simulink model "Coefficients"  (R2024b)
settings: Solver=VariableStepAuto  StartTime=0.0  StopTime=10.0  RelTol=1e-3
values from neighbouring files (symbols this model uses):
  b = params.b    [Aerodynamics_Coefficient.m]    (also in AeroforcesandMoments.m; initACFT_high.m = 21; initACFT_low.m = 21; init_Cessna.m = 10.9728)
  c = params.c    [Aerodynamics_Coefficient.m]    (also in AeroforcesandMoments.m; initACFT_high.m = 2.5; initACFT_low.m = 2.5; init_Cessna.m = 1.49352)
  CD0 = params.CD0    [Aerodynamics_Coefficient.m]    (also in initACFT_high.m = 0.0281; initACFT_low.m = 0.023; init_Cessna.m = 0.027)
  CD_alpha = params.CD_alpha    [Aerodynamics_Coefficient.m]    (also in initACFT_high.m = 0.5157; initACFT_low.m = 0.1318; init_Cessna.m = 0.26)
  CD_elev = params.CD_elev    [Aerodynamics_Coefficient.m]    (also in initACFT_high.m = 0.0178; initACFT_low.m = 0.0178; init_Cessna.m = 0)
  CI_beta = params.CI_beta    [Aerodynamics_Coefficient.m]
  CI_p = params.CI_p    [Aerodynamics_Coefficient.m]
  CI_r = params.CI_r    [Aerodynamics_Coefficient.m]
  CI_rud = params.CI_rud    [Aerodynamics_Coefficient.m]
  CL0 = params.CL0    [Aerodynamics_Coefficient.m]    (also in initACFT_high.m = 0.209; initACFT_low.m = 0.19; init_Cessna.m = 0.307)
  CL_alpha = params.CL_alpha    [Aerodynamics_Coefficient.m]    (also in initACFT_high.m = 8.7491; initACFT_low.m = 6.1879; init_Cessna.m = 4.41)
  CL_elev = params.CL_elev    [Aerodynamics_Coefficient.m]    (also in initACFT_high.m = 0.538; initACFT_low.m = 0.4727; init_Cessna.m = 0.43)
  CL_q = params.CL_q    [Aerodynamics_Coefficient.m]    (also in initACFT_high.m = 4.14; initACFT_low.m = 4.66; init_Cessna.m = 3.9)
  Cm0 = params.Cm0    [Aerodynamics_Coefficient.m]    (also in initACFT_high.m = 0; initACFT_low.m = 0.0133; init_Cessna.m = 0.04)
  Cm_alpha = params.Cm_alpha    [Aerodynamics_Coefficient.m]    (also in initACFT_high.m = -2.4351; initACFT_low.m = -2.0168; init_Cessna.m = -0.613)
  Cm_AlphaDot = params.Cm_AlphaDot    [Aerodynamics_Coefficient.m]    (also in initACFT_high.m = -4.53; initACFT_low.m = -6.76; init_Cessna.m = -7.27)
  Cm_elev = params.Cm_elev    [Aerodynamics_Coefficient.m]    (also in initACFT_high.m = -1.9079; initACFT_low.m = -1.6788; init_Cessna.m = -1.122)
  Cm_q = params.Cm_q    [Aerodynamics_Coefficient.m]    (also in initACFT_high.m = -37.6; initACFT_low.m = -36.3; init_Cessna.m = -12.4)
  Cn_ail = -8.5944e-04    (= -0.00085944)    [initACFT_high.m]    (also in initACFT_low.m = -0.00063025; init_Cessna.m = -0.0216)
  Cn_beta = 0.1478    [initACFT_high.m]    (also in initACFT_low.m = 0.1209; init_Cessna.m = 0.0587)
  Cn_p = -0.114    [initACFT_high.m]    (also in initACFT_low.m; init_Cessna.m = -0.0278)
  Cn_r = -0.15    [initACFT_high.m]    (also in initACFT_low.m = -0.3; init_Cessna.m = -0.0937)
  Cn_rud = -0.1100    (= -0.11)    [initACFT_high.m]    (also in initACFT_low.m = -0.102; init_Cessna.m = -0.0645)
  CY_ail = 0    [initACFT_high.m]    (also in initACFT_low.m; init_Cessna.m)
  CY_beta = params.CY_beta    [Aerodynamics_Coefficient.m]    (also in initACFT_high.m = -1.2777; initACFT_low.m = -1.1803; init_Cessna.m = -0.404)
  CY_p = params.CY_p    [Aerodynamics_Coefficient.m]    (also in initACFT_high.m = 0.3; initACFT_low.m = 0.3; init_Cessna.m = -0.075)
  CY_r = params.CY_r    [Aerodynamics_Coefficient.m]    (also in initACFT_high.m = 0.91; initACFT_low.m = 0.91; init_Cessna.m = 0.214)
  CY_rud = params.CY_rud    [Aerodynamics_Coefficient.m]    (also in initACFT_high.m = 0.4343; initACFT_low.m = 0.4016; init_Cessna.m = 0.187)
  S = 45    [initACFT_high.m]    (also in initACFT_low.m; init_Cessna.m = 16.2)
undefined symbols (not defined in the file or in its folder): CI_ail, CL_AlphaDot_, Y_cg, Z_cg

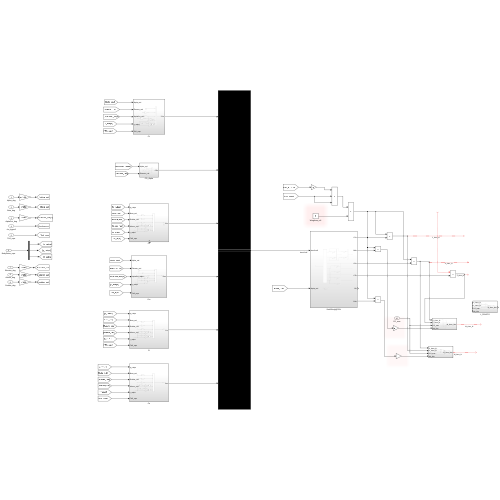
[thumbnail: Simulink's stored preview of the top-level diagram]
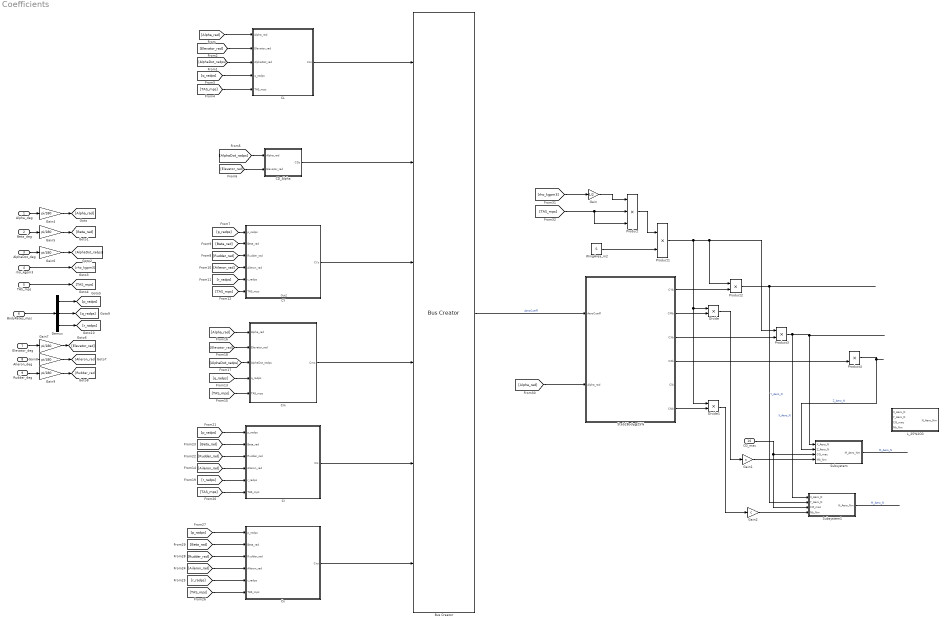
== system Coefficients ==
  Alpha_deg : Inport
  Beta_deg : Inport  Port=2
  AlphaDot_deg : Inport  Port=3
  rho_kgpm3 : Inport  Port=4
  TAS_mps : Inport  Port=5
  BodyRates_mps : Inport  Port=6
  Elevator_deg : Inport  Port=7
  Aileron_deg : Inport  Port=8
  Rudder_deg : Inport  Port=9
  CG_mac : Inport  Port=10
  Bus Creator : BusCreator  Inputs=6
  CD_Alpha : Subsystem
  CI : Subsystem
  CL : Subsystem
  CY : Subsystem
      settings: PortSchema="{\"entries\":[{\"content\":{\"sides\":[{\"content\":{\"connectorIds\":[\"In1\",\"In2\",\"In3\",\"In4\",\"In5\",\"In6\"]},\"type\":\"ConnectorPlacement.EquallySpacedRectSide\",\"uuid\":\"cf27de7d-07f8-4cbf-b6d7-bb20821c77c6\"},{\"content\":{\"connectorIds\":[\"Out1\"],\"side\":\"RIGHT\"},\"type\":\"ConnectorPlacement.EquallySpacedRectSide\",\"uuid\":\"f24d40b1-0b9f-4cab-b37e-a7503e974de5\"},{\"content\":{\"side\":\"TOP\"},\"type\":\"ConnectorPlacement.EquallySpacedRectSide\",\"uuid\":\"b0626d26-2b97-4927-834a-53d4ff987b45\"},{\"content\":{\"connectorIds\":[\"Out2\"],\"side\":\"BOTTOM\"},\"type\":\"ConnectorPlacement.EquallySpacedRectSide\",\"uuid\":\"9cececd4-1f67-47fb-9396-7a7e586ce31d\"}]},\"type\":\"ConnectorPlacement.EquallySpacedConnector\",\"uuid\":\"f6062f6f-5301-4f2b-96bc-d3beb1582379\"}],\"packageUris\":[\"http://schema.mathworks.com/mf0/Connector/R2020b\"],\"version\":\"1.0\"}"
  Cm : Subsystem
  Cn : Subsystem
  Demux : Demux  Outputs=3
  Divide : Product
  Divide1 : Product
  Gain : Gain  Gain=1/2
  Gain1 : Gain  Gain=c
  Gain2 : Gain  Gain=c
  Gain{4..9} (6 alike) : Gain  Gain=pi/180
  L_25%2CG : Subsystem
  Product : Product  Inputs=3
  Product{1..4} (4 alike) : Product
  Stab2Body@25% : Subsystem
  Subsystem : Subsystem
  Subsystem1 : Subsystem
  WingArea_m2 : Constant  Value=S
  wires:
  AlphaDot_deg/1 -> Gain6/1
  rho_kgpm3/1 -> [rho_kgpm3]
  TAS_mps/1 -> [TAS_mps]
  Elevator_deg/1 -> Gain7/1
  Aileron_deg/1 -> Gain8/1
  Rudder_deg/1 -> Gain9/1
  Alpha_deg/1 -> Gain4/1
  Gain4/1 -> [Alpha_rad]
  Beta_deg/1 -> Gain5/1
  Gain5/1 -> [Beta_rad]
  Gain6/1 -> [AlphaDot_radps]
  Gain7/1 -> [Elevator_rad]
  Gain8/1 -> [Aileron_rad]
  Gain9/1 -> [Rudder_rad]
  [Elevator_rad] -> CL/2(Elevator_rad)
  [Alpha_rad] -> CL/1(Alpha_rad)
  [AlphaDot_radps] -> CL/3(AlphaDot_rad)
  [q_radps] -> CL/4(q_radps)
  BodyRates_mps/1 -> Demux/1
  Demux/2 -> [q_radps]
  Demux/1 -> [p_radps]
  Demux/3 -> [r_radps]
  [TAS_mps] -> CL/5(TAS_mps)
  [Elevator_rad] -> CD_Alpha/2(Elevator_rad)
  [AlphaDot_radps] -> CD_Alpha/1(Alpha_rad)
  [p_radps] -> CY/1(p_radps)
  [Rudder_rad] -> CY/3(Rudder_rad)
  [Beta_rad] -> CY/2(Beta_rad)
  [Aileron_rad] -> CY/4(Aileron_rad)
  [r_radps] -> CY/5(r_radps)
  [TAS_mps] -> CY/6(TAS_mps)
  [TAS_mps] -> Cm/5(TAS_mps)
  [Alpha_rad] -> Cm/1(Alpha_rad)
  [Elevator_rad] -> Cm/2(Elevator_rad)
  [AlphaDot_radps] -> Cm/3(AlphaDot_radps)
  [q_radps] -> Cm/4(q_radps)
  [p_radps] -> CI/1(p_radps)
  [Beta_rad] -> CI/2(Beta_rad)
  [Rudder_rad] -> CI/3(Rudder_rad)
  [Aileron_rad] -> CI/4(Aileron_rad)
  [r_radps] -> CI/5(r_radps)
  [TAS_mps] -> CI/6(TAS_mps)
  [TAS_mps] -> Cn/6(TAS_mps)
  [r_radps] -> Cn/5(r_radps)
  [Aileron_rad] -> Cn/4(Aileron_rad)
  [Beta_rad] -> Cn/2(Beta_rad)
  [p_radps] -> Cn/1(p_radps)
  [Rudder_rad] -> Cn/3(Rudder_rad)
  CL/1(CLs) -> Bus Creator/1
  CD_Alpha/1(CDs) -> Bus Creator/2
  CY/1(CYs) -> Bus Creator/3
  Cm/1(Cms) -> Bus Creator/4
  CI/1(CIs) -> Bus Creator/5
  Cn/1(Cns) -> Bus Creator/6
  Bus Creator/1 -> Stab2Body@25%/1(AeroCoeff)  "AeroCoeff"
  [Alpha_rad] -> Stab2Body@25%/2(Alpha_rad)
  [rho_kgpm3] -> Gain/1
  Gain/1 -> Product/1
  [TAS_mps] -> Product/3, Product/2
  WingArea_m2/1 -> Product1/2
  Product/1 -> Product1/1
  Stab2Body@25%/1(CYb) -> Product2/2
  Stab2Body@25%/3(CXb) -> Product3/2
  Stab2Body@25%/4(CZb) -> Product4/2
  Product1/1 -> Divide1/1, Divide/1, Product2/1, Product3/1
  ? -> Product4/1
  Product2/1 -> Subsystem1/2(Y_Aero_N)  "Y_Aero_N"
  Product3/1 -> Subsystem1/1(X_Aero_N), Subsystem/1(X_Aero_N)  "X_Aero_N"
  Product4/1 -> Subsystem/2(Z_Aero_N)  "Z_Aero_N"
  CG_mac/1 -> Subsystem1/3(CG_mac), Subsystem/3(CG_mac)
  Stab2Body@25%/2(CMb) -> Divide/2
  Divide/1 -> Gain1/1
  Subsystem/1(M_Aero_Nm) -> ?  "M_Aero_N"
  Gain1/1 -> Subsystem/4(Mb_Nm)
  Subsystem1/1(N_Aero_Nm) -> ?  "M_Aero_N"
  Stab2Body@25%/6(CNb) -> Divide1/2
  Gain2/1 -> Subsystem1/4(Nb_Nm)
  Divide1/1 -> Gain2/1

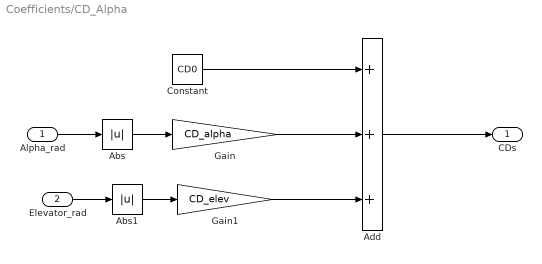
== system Coefficients/CD_Alpha ==
  Alpha_rad : Inport
  Elevator_rad : Inport  Port=2
  Abs : Abs  SaturateOnIntegerOverflow=off
  Abs1 : Abs  SaturateOnIntegerOverflow=off
  Add : Sum  Inputs=+++
  Constant : Constant  Value=CD0
  Gain : Gain  Gain=CD_alpha
  Gain1 : Gain  Gain=CD_elev
  CDs : Outport
  wires:
  Abs1/1 -> Gain1/1
  Alpha_rad/1 -> Abs/1
  Constant/1 -> Add/1
  Abs/1 -> Gain/1
  Add/1 -> CDs/1
  Elevator_rad/1 -> Abs1/1
  Gain1/1 -> Add/3
  Gain/1 -> Add/2

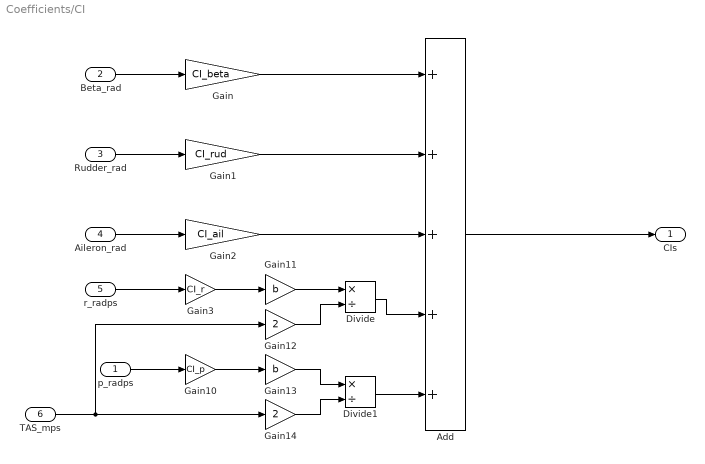
== system Coefficients/CI ==
  p_radps : Inport
  Beta_rad : Inport  Port=2
  Rudder_rad : Inport  Port=3
  Aileron_rad : Inport  Port=4
  r_radps : Inport  Port=5
  TAS_mps : Inport  Port=6
  Add : Sum  Inputs=+++++
  Divide : Product  Inputs=*/
  Divide1 : Product  Inputs=*/
  Gain : Gain  Gain=CI_beta
  Gain1 : Gain  Gain=CI_rud
  Gain10 : Gain  Gain=CI_p
  Gain11 : Gain  Gain=b
  Gain12 : Gain  Gain=2
  Gain13 : Gain  Gain=b
  Gain14 : Gain  Gain=2
  Gain2 : Gain  Gain=CI_ail
  Gain3 : Gain  Gain=CI_r
  CIs : Outport
  wires:
  Gain13/1 -> Divide1/1
  Gain/1 -> Add/1
  Gain3/1 -> Gain11/1
  Rudder_rad/1 -> Gain1/1
  Gain2/1 -> Add/3
  Add/1 -> CIs/1
  Gain12/1 -> Divide/2
  Gain11/1 -> Divide/1
  Gain14/1 -> Divide1/2
  TAS_mps/1 -> Gain12/1, Gain14/1
  Gain10/1 -> Gain13/1
  Divide/1 -> Add/4
  p_radps/1 -> Gain10/1
  Gain1/1 -> Add/2
  Aileron_rad/1 -> Gain2/1
  Beta_rad/1 -> Gain/1
  r_radps/1 -> Gain3/1
  Divide1/1 -> Add/5

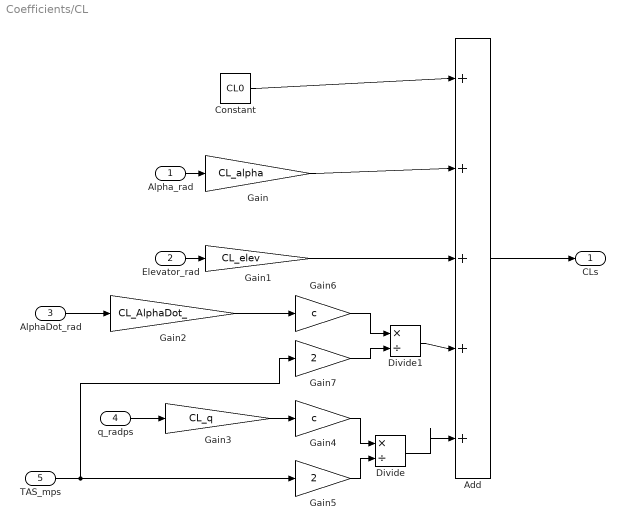
== system Coefficients/CL ==
  Alpha_rad : Inport
  Elevator_rad : Inport  Port=2
  AlphaDot_rad : Inport  Port=3
  q_radps : Inport  Port=4
  TAS_mps : Inport  Port=5
  Add : Sum  Inputs=+++++
  Constant : Constant  Value=CL0
  Divide : Product  Inputs=*/
  Divide1 : Product  Inputs=*/
  Gain : Gain  Gain=CL_alpha
  Gain1 : Gain  Gain=CL_elev
  Gain2 : Gain  Gain=CL_AlphaDot_
  Gain3 : Gain  Gain=CL_q
  Gain4 : Gain  Gain=c
  Gain5 : Gain  Gain=2
  Gain6 : Gain  Gain=c
  Gain7 : Gain  Gain=2
  CLs : Outport
  wires:
  Alpha_rad/1 -> Gain/1
  q_radps/1 -> Gain3/1
  AlphaDot_rad/1 -> Gain2/1
  Gain1/1 -> Add/3
  Elevator_rad/1 -> Gain1/1
  Gain/1 -> Add/2
  Constant/1 -> Add/1
  Gain2/1 -> Gain6/1
  Add/1 -> CLs/1
  Gain3/1 -> Gain4/1
  TAS_mps/1 -> Gain7/1, Gain5/1
  Gain5/1 -> Divide/2
  Divide/1 -> Add/5
  Gain4/1 -> Divide/1
  Gain6/1 -> Divide1/1
  Divide1/1 -> Add/4
  Gain7/1 -> Divide1/2

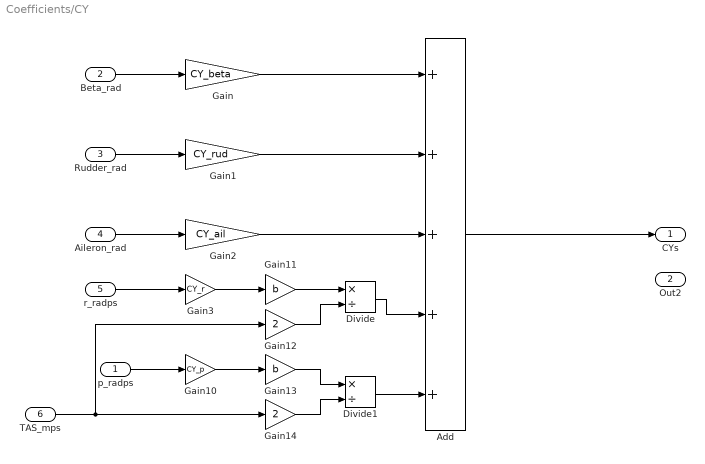
== system Coefficients/CY ==
  p_radps : Inport
  Beta_rad : Inport  Port=2
  Rudder_rad : Inport  Port=3
  Aileron_rad : Inport  Port=4
  r_radps : Inport  Port=5
  TAS_mps : Inport  Port=6
  Add : Sum  Inputs=+++++
  Divide : Product  Inputs=*/
  Divide1 : Product  Inputs=*/
  Gain : Gain  Gain=CY_beta
  Gain1 : Gain  Gain=CY_rud
  Gain10 : Gain  Gain=CY_p
  Gain11 : Gain  Gain=b
  Gain12 : Gain  Gain=2
  Gain13 : Gain  Gain=b
  Gain14 : Gain  Gain=2
  Gain2 : Gain  Gain=CY_ail
  Gain3 : Gain  Gain=CY_r
  CYs : Outport
  Out2 : Outport  Port=2
  wires:
  Gain13/1 -> Divide1/1
  Gain/1 -> Add/1
  Gain3/1 -> Gain11/1
  Rudder_rad/1 -> Gain1/1
  Gain2/1 -> Add/3
  Add/1 -> CYs/1
  Gain12/1 -> Divide/2
  Gain11/1 -> Divide/1
  Gain14/1 -> Divide1/2
  TAS_mps/1 -> Gain12/1, Gain14/1
  Gain10/1 -> Gain13/1
  Divide/1 -> Add/4
  p_radps/1 -> Gain10/1
  Gain1/1 -> Add/2
  Aileron_rad/1 -> Gain2/1
  Beta_rad/1 -> Gain/1
  r_radps/1 -> Gain3/1
  Divide1/1 -> Add/5

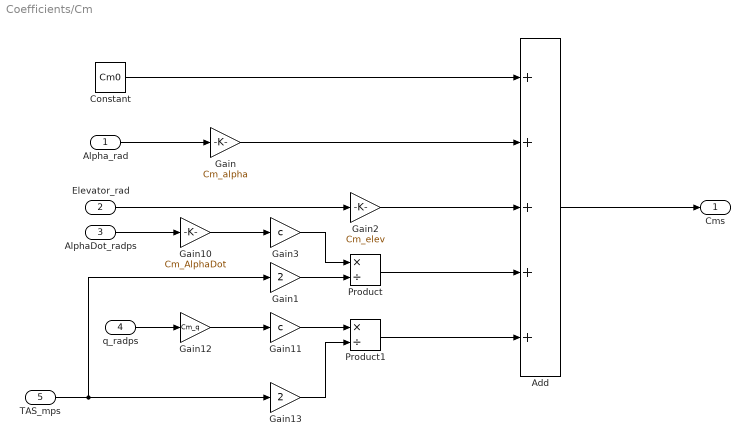
== system Coefficients/Cm ==
  Alpha_rad : Inport
  Elevator_rad : Inport  Port=2
  AlphaDot_radps : Inport  Port=3
  q_radps : Inport  Port=4
  TAS_mps : Inport  Port=5
  Add : Sum  Inputs=+++++
  Constant : Constant  Value=Cm0
  Gain : Gain  Gain=Cm_alpha
  Gain1 : Gain  Gain=2
  Gain10 : Gain  Gain=Cm_AlphaDot
  Gain11 : Gain  Gain=c
  Gain12 : Gain  Gain=Cm_q
  Gain13 : Gain  Gain=2
  Gain2 : Gain  Gain=Cm_elev
  Gain3 : Gain  Gain=c
  Product : Product  Inputs=*/
  Product1 : Product  Inputs=*/
  Cms : Outport
  wires:
  AlphaDot_radps/1 -> Gain10/1
  Elevator_rad/1 -> Gain2/1
  Constant/1 -> Add/1
  TAS_mps/1 -> Gain1/1, Gain13/1
  Gain1/1 -> Product/2
  Gain2/1 -> Add/3
  Alpha_rad/1 -> Gain/1
  Product1/1 -> Add/5
  Gain3/1 -> Product/1
  Gain13/1 -> Product1/2
  Gain12/1 -> Gain11/1
  q_radps/1 -> Gain12/1
  Gain10/1 -> Gain3/1
  Gain11/1 -> Product1/1
  Gain/1 -> Add/2
  Product/1 -> Add/4
  Add/1 -> Cms/1

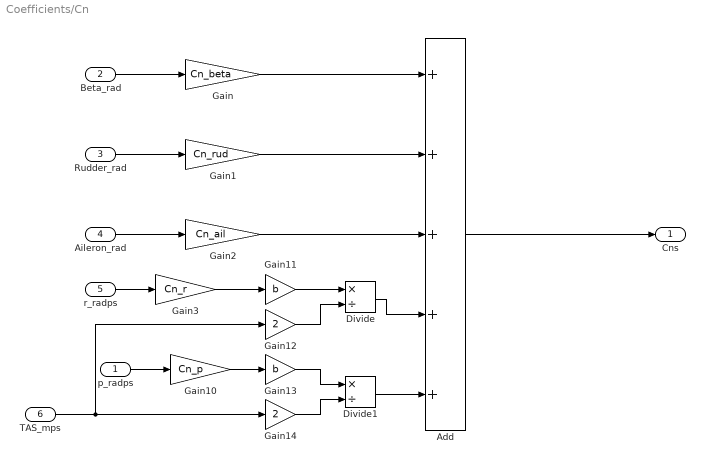
== system Coefficients/Cn ==
  p_radps : Inport
  Beta_rad : Inport  Port=2
  Rudder_rad : Inport  Port=3
  Aileron_rad : Inport  Port=4
  r_radps : Inport  Port=5
  TAS_mps : Inport  Port=6
  Add : Sum  Inputs=+++++
  Divide : Product  Inputs=*/
  Divide1 : Product  Inputs=*/
  Gain : Gain  Gain=Cn_beta
  Gain1 : Gain  Gain=Cn_rud
  Gain10 : Gain  Gain=Cn_p
  Gain11 : Gain  Gain=b
  Gain12 : Gain  Gain=2
  Gain13 : Gain  Gain=b
  Gain14 : Gain  Gain=2
  Gain2 : Gain  Gain=Cn_ail
  Gain3 : Gain  Gain=Cn_r
  Cns : Outport
  wires:
  Gain13/1 -> Divide1/1
  Gain/1 -> Add/1
  Gain3/1 -> Gain11/1
  Rudder_rad/1 -> Gain1/1
  Gain2/1 -> Add/3
  Add/1 -> Cns/1
  Gain12/1 -> Divide/2
  Gain11/1 -> Divide/1
  Gain14/1 -> Divide1/2
  TAS_mps/1 -> Gain12/1, Gain14/1
  Gain10/1 -> Gain13/1
  Divide/1 -> Add/4
  p_radps/1 -> Gain10/1
  Gain1/1 -> Add/2
  Aileron_rad/1 -> Gain2/1
  Beta_rad/1 -> Gain/1
  r_radps/1 -> Gain3/1
  Divide1/1 -> Add/5

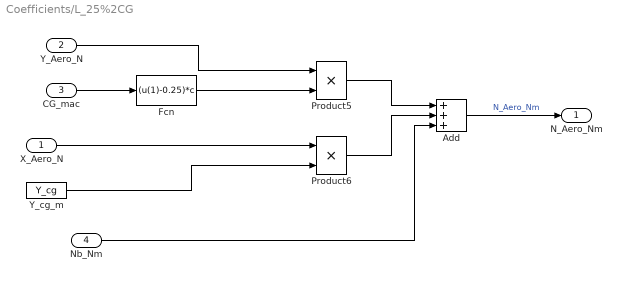
== system Coefficients/L_25%2CG ==
  X_Aero_N : Inport
  Y_Aero_N : Inport  Port=2
  CG_mac : Inport  Port=3
  Nb_Nm : Inport  Port=4
  Add : Sum  Inputs=+++
  Fcn : Fcn  Expr=(u(1)-0.25)*c
  Product5 : Product
  Product6 : Product
  Y_cg_m : Constant  Value=Y_cg
  N_Aero_Nm : Outport
  wires:
  Product6/1 -> Add/2
  CG_mac/1 -> Fcn/1
  Product5/1 -> Add/1
  Y_cg_m/1 -> Product6/2
  Y_Aero_N/1 -> Product5/1
  Fcn/1 -> Product5/2
  X_Aero_N/1 -> Product6/1
  Add/1 -> N_Aero_Nm/1  "N_Aero_Nm"
  Nb_Nm/1 -> Add/3

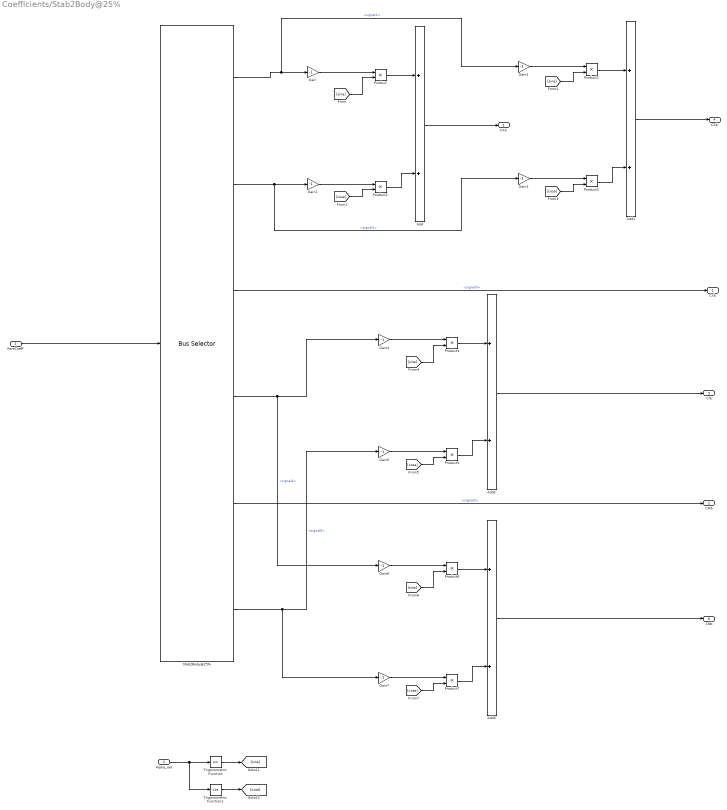
== system Coefficients/Stab2Body@25% ==
  AeroCoeff : Inport
  Alpha_rad : Inport  Port=2
  Add{,1..3} (4 alike) : Sum
  Gain{,1..7} (8 alike) : Gain  Gain=-1
  Product{,1..7} (8 alike) : Product
  Stab2Body@25% : BusSelector  OutputSignals=signal1,signal2,signal3,signal4,signal5,signal6
  Trigonometric Function : Trigonometry
  Trigonometric Function1 : Trigonometry  Operator=cos
  CYb : Outport
  CMb : Outport  Port=2
  CXb : Outport  Port=3
  CZb : Outport  Port=4
  Clb : Outport  Port=5
  CNb : Outport  Port=6
  wires:
  AeroCoeff/1 -> Stab2Body@25%/1
  Stab2Body@25%/5 -> CMb/1  "<signal5>"
  Stab2Body@25%/3 -> CYb/1  "<signal3>"
  Stab2Body@25%/1 -> Gain2/1, Gain/1  "<signal1>"
  Trigonometric Function/1 -> [sina]
  Trigonometric Function1/1 -> [cosa]
  Alpha_rad/1 -> Trigonometric Function1/1, Trigonometric Function/1
  Product/1 -> Add/1
  Product1/1 -> Add/2
  Gain/1 -> Product/1
  Gain1/1 -> Product1/1
  [sina] -> Product/2
  [cosa] -> Product1/2
  Add/1 -> CXb/1
  Product2/1 -> Add1/1
  Gain3/1 -> Product3/1
  [sina] -> Product2/2
  Add1/1 -> CZb/1
  Product3/1 -> Add1/2
  Gain2/1 -> Product2/1
  Stab2Body@25%/2 -> Gain3/1, Gain1/1  "<signal2>"
  [cosa] -> Product3/2
  Product4/1 -> Add2/1
  Gain5/1 -> Product5/1
  [sina] -> Product4/2
  Add2/1 -> Clb/1
  Stab2Body@25%/6 -> Gain7/1, Gain5/1  "<signal6>"
  Product5/1 -> Add2/2
  Stab2Body@25%/4 -> Gain6/1, Gain4/1  "<signal4>"
  Gain4/1 -> Product4/1
  [cosa] -> Product5/2
  [sina] -> Product6/2
  Gain6/1 -> Product6/1
  [cosa] -> Product7/2
  Gain7/1 -> Product7/1
  Add3/1 -> CNb/1
  Product6/1 -> Add3/1
  Product7/1 -> Add3/2

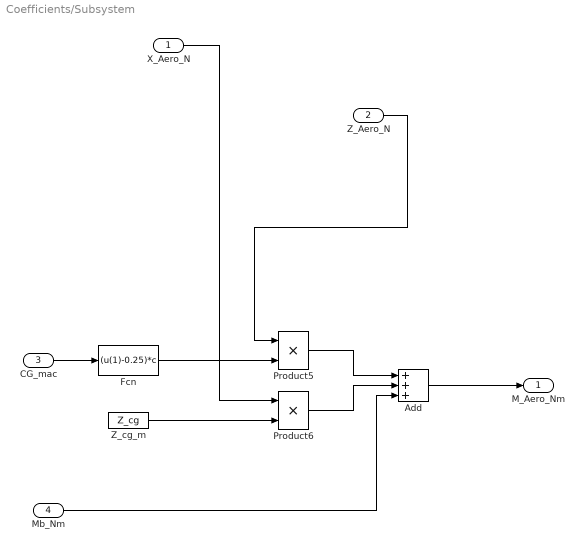
== system Coefficients/Subsystem ==
  X_Aero_N : Inport
  Z_Aero_N : Inport  Port=2
  CG_mac : Inport  Port=3
  Mb_Nm : Inport  Port=4
  Add : Sum  Inputs=+++
  Fcn : Fcn  Expr=(u(1)-0.25)*c
  Product5 : Product
  Product6 : Product
  Z_cg_m : Constant  Value=Z_cg
  M_Aero_Nm : Outport
  wires:
  Product6/1 -> Add/2
  CG_mac/1 -> Fcn/1
  Product5/1 -> Add/1
  Z_cg_m/1 -> Product6/2
  Z_Aero_N/1 -> Product5/1
  Fcn/1 -> Product5/2
  X_Aero_N/1 -> Product6/1
  Add/1 -> M_Aero_Nm/1
  Mb_Nm/1 -> Add/3

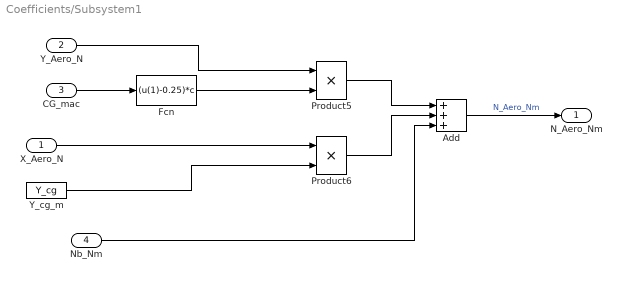
== system Coefficients/Subsystem1 ==
  X_Aero_N : Inport
  Y_Aero_N : Inport  Port=2
  CG_mac : Inport  Port=3
  Nb_Nm : Inport  Port=4
  Add : Sum  Inputs=+++
  Fcn : Fcn  Expr=(u(1)-0.25)*c
  Product5 : Product
  Product6 : Product
  Y_cg_m : Constant  Value=Y_cg
  N_Aero_Nm : Outport
  wires:
  Product6/1 -> Add/2
  CG_mac/1 -> Fcn/1
  Product5/1 -> Add/1
  Y_cg_m/1 -> Product6/2
  Y_Aero_N/1 -> Product5/1
  Fcn/1 -> Product5/2
  X_Aero_N/1 -> Product6/1
  Add/1 -> N_Aero_Nm/1  "N_Aero_Nm"
  Nb_Nm/1 -> Add/3
